simulink model "BP_PID"  (R2018b)
settings: Solver=FixedStepAuto  StartTime=0.0  StopTime=200  FixedStep=0.01  RelTol=1e-3
settings Model: Creator=Administrator  LastModifiedBy=time
settings SFSimCC: SimUseLocalCustomCode=off
settings RTWCC: RTWUseLocalCustomCode=off
settings CodeAppCC: StateflowObjectComments=on

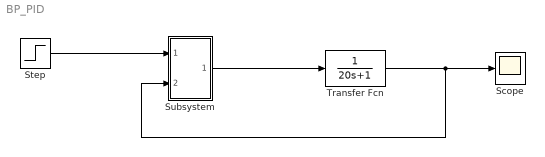
== system BP_PID ==
  Scope : Scope
  Step : Step  SampleTime=0.01
  Subsystem : Subsystem
  Transfer Fcn : TransferFcn  Denominator=[20 1]
  wires:
  Step/1 -> Subsystem/1(r(k))
  Subsystem/1(u(k)) -> Transfer Fcn/1
  Transfer Fcn/1 -> Subsystem/2(y(k)), Scope/1

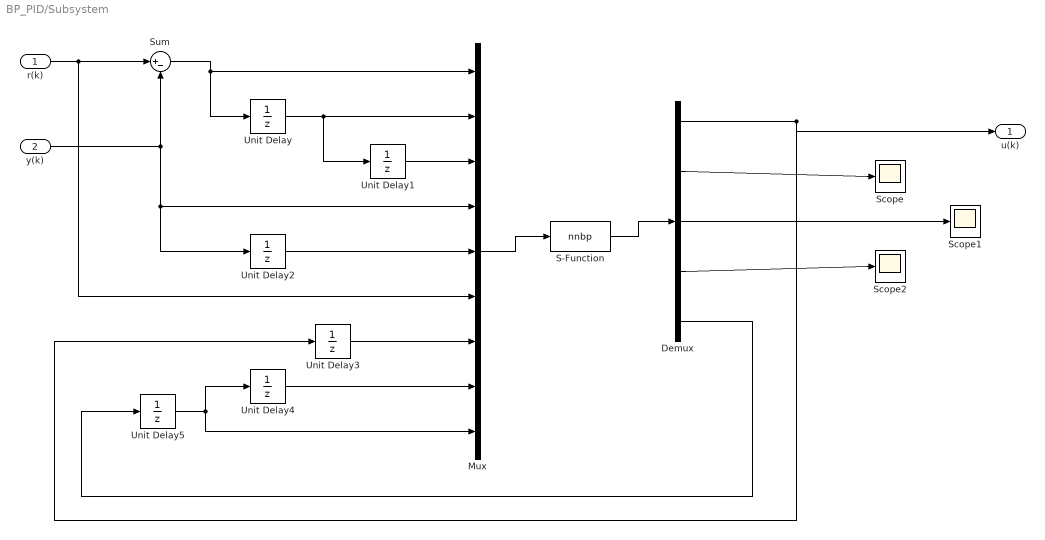
== system BP_PID/Subsystem ==
  r(k) : Inport
  y(k) : Inport  Port=2
  Demux : Demux  Outputs=[1 1 1 1 48]
  Mux : Mux  Inputs=[1 1 1 1 1 1 1 48 48]
  S-Function : S-Function  FunctionName=nnbp  Parameters=T,nh,xite,alfa  SFunctionDeploymentMode=off  EnableBusSupport=off  mask{T=0.01, nh=8, xite=0.3, alfa=0.3}
  Scope : Scope
  Scope1 : Scope
  Scope2 : Scope
  Sum : Sum  Inputs=|+-
  Unit Delay{,1..5} (6 alike) : UnitDelay  SampleTime=-1
  u(k) : Outport
  wires:
  r(k)/1 -> Mux/6, Sum/1
  Sum/1 -> Mux/1, Unit Delay/1
  Unit Delay/1 -> Mux/2, Unit Delay1/1
  Unit Delay1/1 -> Mux/3
  y(k)/1 -> Unit Delay2/1, Mux/4, Sum/2
  Unit Delay2/1 -> Mux/5
  Unit Delay3/1 -> Mux/7
  Unit Delay4/1 -> Mux/8
  Unit Delay5/1 -> Mux/9, Unit Delay4/1
  Mux/1 -> S-Function/1
  S-Function/1 -> Demux/1
  Demux/1 -> Unit Delay3/1, u(k)/1
  Demux/2 -> Scope/1
  Demux/3 -> Scope1/1
  Demux/4 -> Scope2/1
  Demux/5 -> Unit Delay5/1
